simulink model "symulink_one"  (R2020a)
settings: Solver=VariableStepAuto  StartTime=0.0  StopTime=4  RelTol=1e-3
settings Model: Creator=dinossaurobebado  LastModifiedBy=dinossaurobebado

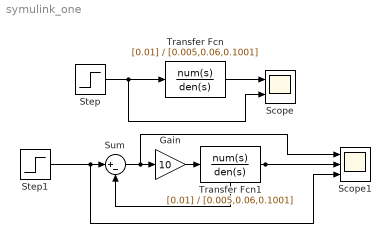
== system symulink_one ==
  Gain : Gain  Gain=10
  Scope : Scope  NumInputPorts=2
  Scope1 : Scope  NumInputPorts=3
  Step : Step  SampleTime=0
  Step1 : Step  SampleTime=0
  Sum : Sum  Inputs=|+-
  Transfer Fcn : TransferFcn  Numerator=[0.01]  Denominator=[0.005,0.06,0.1001]  ContinuousStateAttributes='pos'
  Transfer Fcn1 : TransferFcn  Numerator=[0.01]  Denominator=[0.005,0.06,0.1001]  ContinuousStateAttributes='pos'
  wires:
  Step/1 -> Scope/2, Transfer Fcn/1
  Transfer Fcn/1 -> Scope/1
  Transfer Fcn1/1 -> Sum/2, Scope1/2
  Step1/1 -> Scope1/3, Sum/1
  Gain/1 -> Transfer Fcn1/1
  Sum/1 -> Scope1/1, Gain/1
